simulink model "Chua_"  (R2019a)
settings: Solver=VariableStepAuto  StartTime=0.0  StopTime=100  RelTol=1e-3
libraries: simulink x2
settings Model: Creator=DELL  LastModifiedBy=DELL

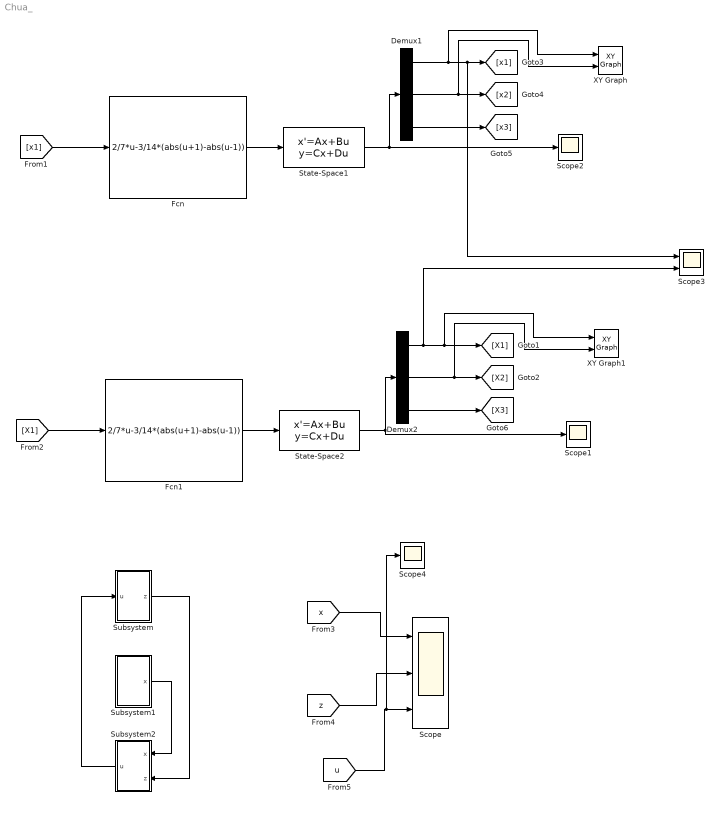
== system Chua_ ==
  Demux1 : Demux  Outputs=3
  Demux2 : Demux  Outputs=3
  Fcn : Fcn  Expr=2/7*u-3/14*(abs(u+1)-abs(u-1))
  Fcn1 : Fcn  Expr=2/7*u-3/14*(abs(u+1)-abs(u-1))
  Scope : Scope  NumInputPorts=3
  Scope1 : Scope
  Scope2 : Scope
  Scope3 : Scope  NumInputPorts=2
  Scope4 : Scope
  State-Space1 : StateSpace  A=[0 9 0;1 -1 1;0 -14.28 0]  B=[-9;0;0]  C=[1 0 0;0 1 0;0 0 1]  D=[0;0;0]  InitialCondition=[-0.2;0.3;0.7]
  State-Space2 : StateSpace  A=[0 9 0;1 -1 1;0 -14.28 0]  B=[-9;0;0]  C=[1 0 0;0 1 0;0 0 1]  D=[0;0;0]  InitialCondition=[0.2;0.5;0.9]
  Subsystem : Subsystem
  Subsystem1 : Subsystem
  Subsystem2 : Subsystem
  XY Graph : simulink/Sinks/XY Graph  xmin=-2.5  xmax=2.5  ymin=-1  ymax=1  st=-1
  XY Graph1 : simulink/Sinks/XY Graph  xmin=-2.5  xmax=2.5  ymin=-1  ymax=1  st=-1
  wires:
  Demux1/2 -> XY Graph/2, [x2]
  Demux1/3 -> [x3]
  Fcn/1 -> State-Space1/1
  [x1] -> Fcn/1
  State-Space1/1 -> Scope2/1, Demux1/1
  Demux1/1 -> XY Graph/1, Scope3/1, [x1]
  Fcn1/1 -> State-Space2/1
  Demux2/2 -> XY Graph1/2, [X2]
  State-Space2/1 -> Scope1/1, Demux2/1
  [X1] -> Fcn1/1
  Demux2/3 -> [X3]
  Demux2/1 -> Scope3/2, XY Graph1/1, [X1]
  Subsystem2/1(u) -> Subsystem/1(u)
  Subsystem1/1(x) -> Subsystem2/1(x)
  Subsystem/1(z) -> Subsystem2/2(z)
  [x] -> Scope/1
  [z] -> Scope/2
  [u] -> Scope4/1, Scope/3

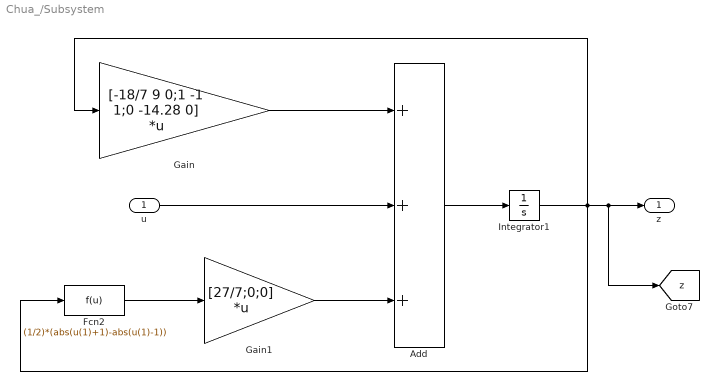
== system Chua_/Subsystem ==
  u : Inport
  Add : Sum  Inputs=+++
  Fcn2 : Fcn  Expr=(1/2)*(abs(u(1)+1)-abs(u(1)-1))
  Gain : Gain  Gain=[-18/7 9 0;1 -1 1;0 -14.28 0]  Multiplication=Matrix(K*u)
  Gain1 : Gain  Gain=[27/7;0;0]  Multiplication=Matrix(K*u)
  Integrator1 : Integrator  InitialCondition=[0.1 0.1 0.1]
  z : Outport
  tag scope: z=global
  wires:
  Gain/1 -> Add/1
  Fcn2/1 -> Gain1/1
  Gain1/1 -> Add/3
  Add/1 -> Integrator1/1
  Integrator1/1 -> Gain/1, Fcn2/1, z/1, [z]
  u/1 -> Add/2

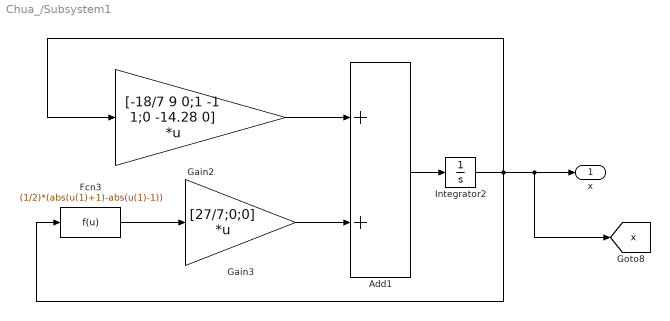
== system Chua_/Subsystem1 ==
  Add1 : Sum
  Fcn3 : Fcn  Expr=(1/2)*(abs(u(1)+1)-abs(u(1)-1))
  Gain2 : Gain  Gain=[-18/7 9 0;1 -1 1;0 -14.28 0]  Multiplication=Matrix(K*u)
  Gain3 : Gain  Gain=[27/7;0;0]  Multiplication=Matrix(K*u)
  Integrator2 : Integrator  InitialCondition=[0.1 0.1 0.1]*3
  x : Outport
  tag scope: x=global
  wires:
  Gain3/1 -> Add1/2
  Integrator2/1 -> Gain2/1, Fcn3/1, x/1, [x]
  Fcn3/1 -> Gain3/1
  Gain2/1 -> Add1/1
  Add1/1 -> Integrator2/1

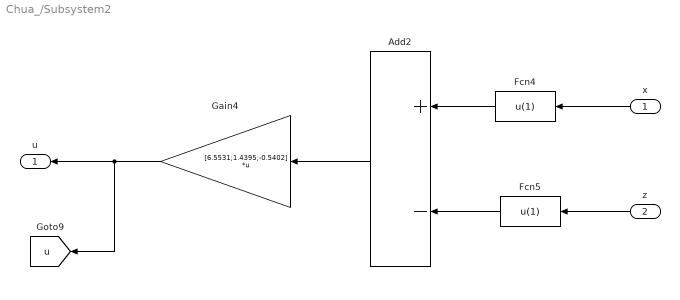
== system Chua_/Subsystem2 ==
  x : Inport
  z : Inport  Port=2
  Add2 : Sum  Inputs=+-
  Fcn4 : Fcn  Expr=u(1)
  Fcn5 : Fcn  Expr=u(1)
  Gain4 : Gain  Gain=[6.5531;1.4395;-0.5402]  Multiplication=Matrix(K*u)
  u : Outport
  tag scope: u=global
  wires:
  Fcn5/1 -> Add2/2
  Add2/1 -> Gain4/1
  z/1 -> Fcn5/1
  x/1 -> Fcn4/1
  Gain4/1 -> u/1, [u]
  Fcn4/1 -> Add2/1
